simulink model "simulation"  (R2022b)
settings: Solver=VariableStepAuto  StartTime=0.0  StopTime=30  RelTol=1e-3
undefined symbols (not defined in the file or in its folder): A_lin_num, B_lin_num, K
settings Model: Creator=Lyn20  LastModifiedBy=Lyn20

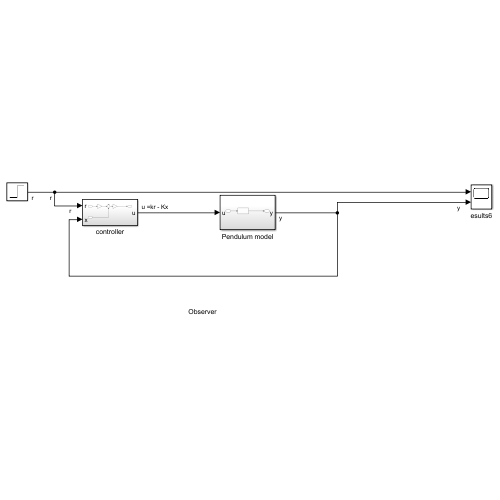
[thumbnail: Simulink's stored preview of the top-level diagram]
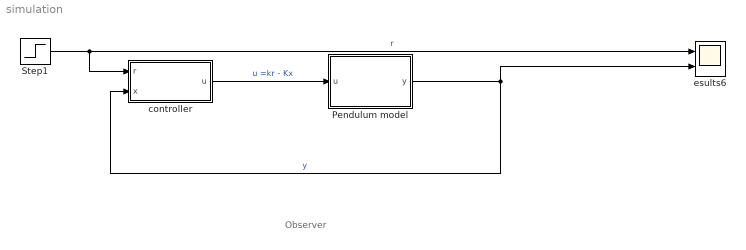
== system simulation ==
  note: Observer
  Pendulum model : Subsystem
  Step1 : Step  Time=5  After=10  SampleTime=0
  controller : Subsystem
  esults6 : Scope  NumInputPorts=2
  wires:
  Step1/1 -> controller/1(r), esults6/1  "r"
  Pendulum model/1(y) -> controller/2(x), esults6/2  "y"
  controller/1(u) -> Pendulum model/1(u)  "u =kr - Kx"

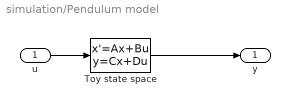
== system simulation/Pendulum model ==
  u : Inport
  Toy state space : StateSpace  A=A_lin_num  B=B_lin_num  C=eye(6)  D=[0,0;0,0;0,0;0,0;0,0;0,0]  InitialCondition=[0.5;0;0;0;0;0]
  y : Outport
  wires:
  u/1 -> Toy state space/1
  Toy state space/1 -> y/1

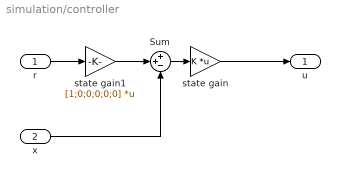
== system simulation/controller ==
  r : Inport
  x : Inport  Port=2
  Sum : Sum  Inputs=++-
  state gain : Gain  Gain=K  Multiplication=Matrix(K*u)
  state gain1 : Gain  Gain=[1;0;0;0;0;0]  Multiplication=Matrix(K*u)
  u : Outport
  wires:
  x/1 -> Sum/3
  r/1 -> state gain1/1
  Sum/1 -> state gain/1
  state gain1/1 -> Sum/2
  state gain/1 -> u/1
